simulink model "req13A"  (R2019a)
settings: Solver=FixedStepAuto  StartTime=0.0  StopTime=100  RelTol=1e-3
libraries: simulink x3
settings Model: Creator=e40014285  LastModifiedBy=e40014285
settings ConfigComp: CovScope=ReferencedModels  CovHTMLOptions=-sRT=1 -sVT=0 -aTS=1 -bRG=1 -bTC=1 -hTR=0 -nFC=0 -nFD=1 -scm=1 -bcm=1 -xEv=0 -xEM=0  CovHtmlReporting=on  CovCumulativeReport=on  DVMaxProcessTime=6000  DVModelCoverageObjectives=EnhancedMCDC  DVTestSuiteOptimization=Auto  DVDetectOutOfBounds=on  DVReportPDFFormat=on  DVRebuildModelRepresentation=Always

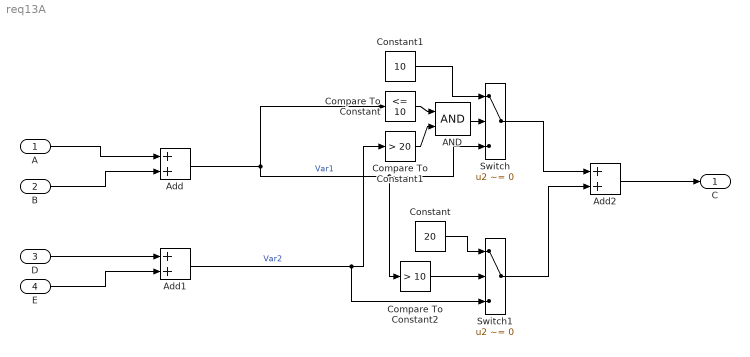
== system req13A ==
  A : Inport
  B : Inport  Port=2
  D : Inport  Port=3
  E : Inport  Port=4
  AND : Logic  AllPortsSameDT=off  OutDataTypeStr=boolean
  Add : Sum
  Add1 : Sum
  Add2 : Sum
  Compare To Constant : simulink/Logic and Bit Operations/Compare To Constant  relop=<=  const=10  OutDataTypeStr=boolean
  Compare To Constant1 : simulink/Logic and Bit Operations/Compare To Constant  relop=>  const=20  OutDataTypeStr=boolean
  Compare To Constant2 : simulink/Logic and Bit Operations/Compare To Constant  relop=>  const=10  OutDataTypeStr=boolean
  Constant : Constant  Value=20
  Constant1 : Constant  Value=10
  Switch : Switch  Criteria=u2 ~= 0
  Switch1 : Switch  Criteria=u2 ~= 0
  C : Outport
  wires:
  Add2/1 -> C/1
  A/1 -> Add/1
  B/1 -> Add/2
  D/1 -> Add1/1
  E/1 -> Add1/2
  Add/1 -> Compare To Constant2/1, Switch/3, Compare To Constant/1  "Var1"
  Add1/1 -> Switch1/3, Compare To Constant1/1  "Var2"
  Constant/1 -> Switch1/1
  AND/1 -> Switch/2
  Compare To Constant/1 -> AND/1
  Compare To Constant1/1 -> AND/2
  Constant1/1 -> Switch/1
  Switch/1 -> Add2/1
  Compare To Constant2/1 -> Switch1/2
  Switch1/1 -> Add2/2
